simulink model "QuadTank_MPC"  (Simulink 6.2)
settings: Solver=ode45  StartTime=0.0  StopTime=1500  RelTol=1e-3
values from neighbouring files (symbols this model uses):
  a1 = 0.071    [Simulate_QT_Simulink_MPC.m]    (also in Simulate_QuadTank_MPC.m)
  A1 = 28    [Simulate_QT_Simulink_MPC.m]    (also in Simulate_QuadTank_MPC.m)
  a2 = 0.057    [Simulate_QT_Simulink_MPC.m]    (also in Simulate_QuadTank_MPC.m)
  A2 = 32    [Simulate_QT_Simulink_MPC.m]    (also in Simulate_QuadTank_MPC.m)
  a3 = 0.071    [Simulate_QT_Simulink_MPC.m]    (also in Simulate_QuadTank_MPC.m)
  A3 = 28    [Simulate_QT_Simulink_MPC.m]    (also in Simulate_QuadTank_MPC.m)
  a4 = 0.057    [Simulate_QT_Simulink_MPC.m]    (also in Simulate_QuadTank_MPC.m)
  A4 = 32    [Simulate_QT_Simulink_MPC.m]    (also in Simulate_QuadTank_MPC.m)
  g = 981    [Simulate_QT_Simulink_MPC.m]    (also in Simulate_QuadTank_MPC.m)
  g1_nmp = 0.25    [Simulate_QT_Simulink_MPC.m]    (also in Simulate_QuadTank_MPC.m)
  g2_nmp = 0.35    [Simulate_QT_Simulink_MPC.m]    (also in Simulate_QuadTank_MPC.m)
  h10_nmp = 8.24441415257276    (= 8.24441415257)    [Simulate_QT_Simulink_MPC.m]    (also in Simulate_QuadTank_MPC.m)
  h20_nmp = 19.01629576919927    (= 19.0162957692)    [Simulate_QT_Simulink_MPC.m]    (also in Simulate_QuadTank_MPC.m)
  h30_nmp = 4.31462580236556    (= 4.31462580237)    [Simulate_QT_Simulink_MPC.m]    (also in Simulate_QuadTank_MPC.m)
  h40_nmp = 8.80652939083585    (= 8.80652939084)    [Simulate_QT_Simulink_MPC.m]    (also in Simulate_QuadTank_MPC.m)
  k1_nmp = 3.33    [Simulate_QT_Simulink_MPC.m]    (also in Simulate_QuadTank_MPC.m)
  k2_nmp = 3.35    [Simulate_QT_Simulink_MPC.m]    (also in Simulate_QuadTank_MPC.m)
  kc = 0.5    [Simulate_QT_Simulink_MPC.m]    (also in Simulate_QuadTank_MPC.m)
  md = MPCInit(Ad,Bd,Cyd,Czd,Dzd,Ccd,Dcd,Hp,Hw,zblk,Hu,ublk,  	    du_max,du_min,u_max,u_min,z_max,  	    z_min,Q,R,W,V,h,4,'qp_as')    [Simulate_QT_Simulink_MPC.m]    (also in Simulate_QuadTank_MPC.m)
  v10_nmp = 3.00    (= 3)    [Simulate_QT_Simulink_MPC.m]    (also in Simulate_QuadTank_MPC.m)
  v20_nmp = 3.00    (= 3)    [Simulate_QT_Simulink_MPC.m]    (also in Simulate_QuadTank_MPC.m)
undefined symbols (not defined in the file or in its folder): QuadTank
settings Model: Creator=jakesson  LastModifiedBy=jakesson  ExtModeAutoUpdateStatusClock=off
settings DataIOCC: SignalLoggingName=sigsOut
settings OptimizationCC: BooleanDataType=off
settings HardwareCC: TargetUnknown=on

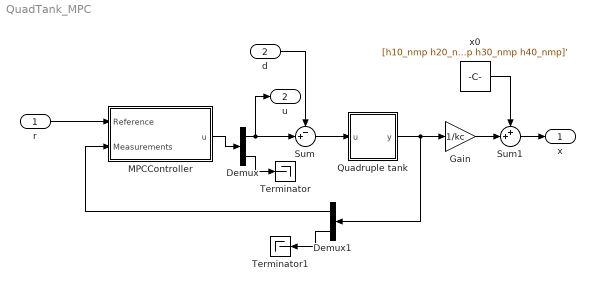
== system QuadTank_MPC ==
  r : Inport  Port=1  LatchInput=off
  d : Inport  Port=2  PortDimensions=2  LatchInput=off
  Demux : Demux  Outputs=[md.m md.ne]
  Demux1 : Demux  Orientation=left  Outputs=[2 2]
  Gain : Gain  Gain=1/kc  SaturateOnIntegerOverflow=on
  MPCController : Subsystem  mask{md=md}
      mask prompts: md "MPCData"
  Quadruple tank : Subsystem
  Sum : Sum  Inputs=-+|  SaturateOnIntegerOverflow=on  InputSameDT=on
  Sum1 : Sum  Inputs=++|  SaturateOnIntegerOverflow=on  InputSameDT=on
  Terminator : Terminator
  Terminator1 : Terminator
  x0 : Constant  Value=[h10_nmp h20_nmp h30_nmp h40_nmp]'
  x : Outport
  u : Outport  Port=2
  wires:
  MPCController/1(u) -> Demux/1
  Sum/1 -> Quadruple tank/1(u)
  d/1 -> Sum/1
  Demux/1 -> Sum/2, u/1
  r/1 -> MPCController/1(Reference)
  Quadruple tank/1(y) -> Gain/1, Demux1/1
  Demux/2 -> Terminator/1
  Demux1/2 -> Terminator1/1
  Sum1/1 -> x/1
  Gain/1 -> Sum1/2
  x0/1 -> Sum1/1
  Demux1/1 -> MPCController/2(Measurements)

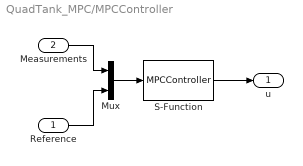
== system QuadTank_MPC/MPCController ==
  Reference : Inport  Port=1  LatchInput=off
  Measurements : Inport  Port=2  LatchInput=off
  Mux : Mux  Inputs=2
  S-Function : S-Function  FunctionName=MPCController  Parameters=md
  u : Outport
  wires:
  Mux/1 -> S-Function/1
  Measurements/1 -> Mux/1
  Reference/1 -> Mux/2
  S-Function/1 -> u/1

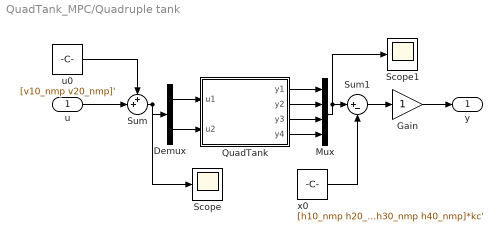
== system QuadTank_MPC/Quadruple tank ==
  u : Inport  Port=1  LatchInput=off
  Demux : Demux  Outputs=2
  Gain : Gain  SaturateOnIntegerOverflow=on
  Mux : Mux
  QuadTank : Subsystem  AncestorBlock=QuadTank/QuadTank  mask{h0=[h10_nmp h20_nmp h30_nmp h40_nmp]', g1=g1_nmp, g2=g2_nmp, k1=k1_nmp, k2=k2_nmp}
      mask prompts: h0 "Initial levels"; g1 "Valve 1"; g2 "Valve 2"; k1 "Pump coefficient 1"; k2 "Pump coefficient 2"
  Scope : Scope
      settings: YMin=-2.5  YMax=17.5  SaveName=ScopeData2
  Scope1 : Scope
      settings: YMin=2  YMax=10  SaveName=ScopeData3
  Sum : Sum  Inputs=++|  SaturateOnIntegerOverflow=on  InputSameDT=on
  Sum1 : Sum  Inputs=|+-  SaturateOnIntegerOverflow=on  InputSameDT=on
  u0 : Constant  Value=[v10_nmp v20_nmp]'
  x0 : Constant  Value=[h10_nmp h20_nmp h30_nmp h40_nmp]*kc'
  y : Outport
  wires:
  Mux/1 -> Scope1/1, Sum1/1
  Sum1/1 -> Gain/1
  x0/1 -> Sum1/2
  u/1 -> Sum/2
  u0/1 -> Sum/1
  Sum/1 -> Scope/1, Demux/1
  QuadTank/2(y2) -> Mux/2
  QuadTank/1(y1) -> Mux/1
  Demux/2 -> QuadTank/2(u2)
  Demux/1 -> QuadTank/1(u1)
  Gain/1 -> y/1
  QuadTank/3(y3) -> Mux/3
  QuadTank/4(y4) -> Mux/4

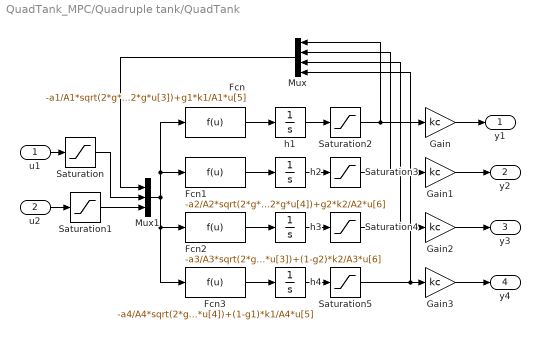
== system QuadTank_MPC/Quadruple tank/QuadTank ==
  u1 : Inport  Port=1  LatchInput=off
  u2 : Inport  Port=2  LatchInput=off
  Fcn : Fcn  Expr=-a1/A1*sqrt(2*g*u[1])+a3/A1*sqrt(2*g*u[3])+g1*k1/A1*u[5]
  Fcn1 : Fcn  Expr=-a2/A2*sqrt(2*g*u[2])+a4/A2*sqrt(2*g*u[4])+g2*k2/A2*u[6]
  Fcn2 : Fcn  Expr=-a3/A3*sqrt(2*g*u[3])+(1-g2)*k2/A3*u[6]
  Fcn3 : Fcn  Expr=-a4/A4*sqrt(2*g*u[4])+(1-g1)*k1/A4*u[5]
  Gain{,1..3} (4 alike) : Gain  Gain=kc  SaturateOnIntegerOverflow=on
  Mux : Mux  Orientation=left
  Mux1 : Mux  Inputs=3
  Saturation : Saturate  UpperLimit=10  LowerLimit=0
  Saturation1 : Saturate  UpperLimit=10  LowerLimit=0
  Saturation{2..5} (4 alike) : Saturate  UpperLimit=50  LowerLimit=0
  h1 : Integrator  InitialCondition=h0(1)
  h2 : Integrator  InitialCondition=h0(2)
  h3 : Integrator  InitialCondition=h0(3)
  h4 : Integrator  InitialCondition=h0(4)
  y1 : Outport
  y2 : Outport  Port=2
  y3 : Outport  Port=3
  y4 : Outport  Port=4
  wires:
  Mux1/1 -> Fcn3/1, Fcn2/1, Fcn1/1, Fcn/1
  Fcn3/1 -> h4/1
  Fcn2/1 -> h3/1
  Fcn1/1 -> h2/1
  Fcn/1 -> h1/1
  u2/1 -> Saturation1/1
  u1/1 -> Saturation/1
  Mux/1 -> Mux1/1
  h2/1 -> Saturation3/1
  h1/1 -> Saturation2/1
  h3/1 -> Saturation4/1
  h4/1 -> Saturation5/1
  Gain3/1 -> y4/1
  Gain2/1 -> y3/1
  Gain1/1 -> y2/1
  Gain/1 -> y1/1
  Saturation/1 -> Mux1/2
  Saturation1/1 -> Mux1/3
  Saturation2/1 -> Mux/1, Gain/1
  Saturation3/1 -> Mux/2, Gain1/1
  Saturation4/1 -> Mux/3, Gain2/1
  Saturation5/1 -> Mux/4, Gain3/1
